simulink model "wave_4"  (Simulink 7.4)
settings: Solver=ode23tb  StartTime=0.0  StopTime=.5  RelTol=1e-3
PreLoadFcn:
  | load gauss_fir;  % pulse shaping coefficients
InitFcn:
  | Ts=1e-4;    % set this to control simulation speed, mainly for wave visualization
  | Line_Length=0.05; % meters
libraries: powerlib x208, simulink x2, dspsrcs4 x1
(part 2 of 2)

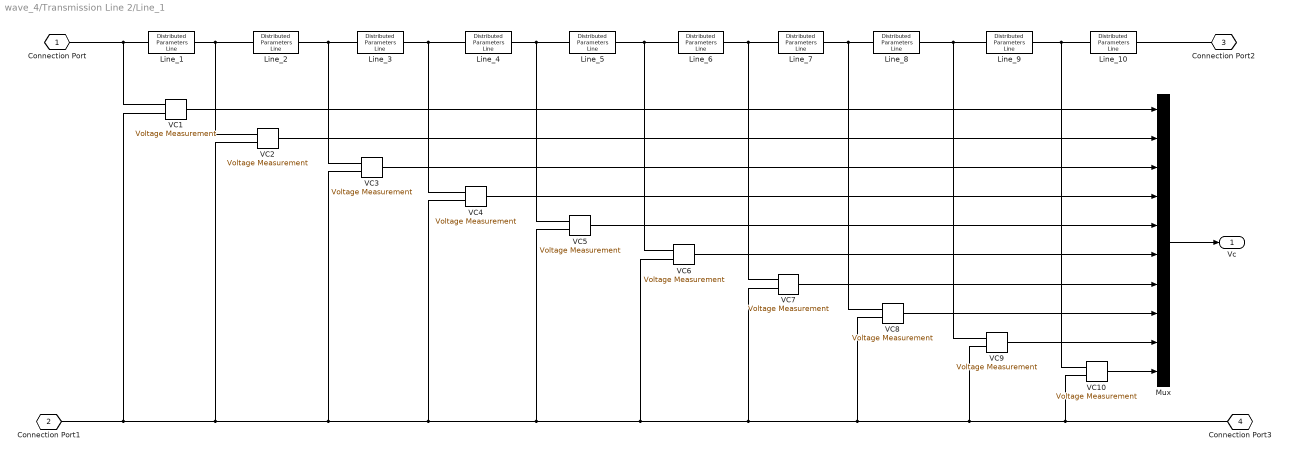
== system wave_4/Transmission Line 2/Line_1 ==
  Line_1 : powerlib/Elements/Distributed Parameters Line  DialogController=POWERSYS.PowerSysDialog  SystemSampleTime=-1  Phases=1  Frequency=60  Resistance=R(1)*1000  Inductance=L(1)*1000  Capacitance=C(1)*1000  Length=Len/(10*1000); % 10 sections in this subsystem  x1=[0 0;0.0002 0;0.0004 0;0.0006 0;0.0008 0;0.001 0]  x2=[0 0;0.0002 0;0.0004 0;0.0006 0;0.0008 0;0.001 0]  x3=[0 0;0.0002 0;0.0004 0;0.0006 0;0.0008 0;0.001 0]  x4=[0 0;0.0002 0;0.0004 0;0.0006 0;0.0008 0;0.001 0]  x5=0.001  Measurements=None
  Line_10 : powerlib/Elements/Distributed Parameters Line  DialogController=POWERSYS.PowerSysDialog  SystemSampleTime=-1  Phases=1  Frequency=60  Resistance=R(10)*1000  Inductance=L(10)*1000  Capacitance=C(10)*1000  Length=Len/(10*1000); % 10 sections in this subsystem  x1=[0 0;0.0002 0;0.0004 0;0.0006 0;0.0008 0;0.001 0]  x2=[0 0;0.0002 0;0.0004 0;0.0006 0;0.0008 0;0.001 0]  x3=[0 0;0.0002 0;0.0004 0;0.0006 0;0.0008 0;0.001 0]  x4=[0 0;0.0002 0;0.0004 0;0.0006 0;0.0008 0;0.001 0]  x5=0.001  Measurements=None
  Line_2 : powerlib/Elements/Distributed Parameters Line  DialogController=POWERSYS.PowerSysDialog  SystemSampleTime=-1  Phases=1  Frequency=60  Resistance=R(2)*1000  Inductance=L(2)*1000  Capacitance=C(2)*1000  Length=Len/(10*1000); % 10 sections in this subsystem  x1=[0 0;0.0002 0;0.0004 0;0.0006 0;0.0008 0;0.001 0]  x2=[0 0;0.0002 0;0.0004 0;0.0006 0;0.0008 0;0.001 0]  x3=[0 0;0.0002 0;0.0004 0;0.0006 0;0.0008 0;0.001 0]  x4=[0 0;0.0002 0;0.0004 0;0.0006 0;0.0008 0;0.001 0]  x5=0.001  Measurements=None
  Line_3 : powerlib/Elements/Distributed Parameters Line  DialogController=POWERSYS.PowerSysDialog  SystemSampleTime=-1  Phases=1  Frequency=60  Resistance=R(3)*1000  Inductance=L(3)*1000  Capacitance=C(3)*1000  Length=Len/(10*1000); % 10 sections in this subsystem  x1=[0 0;0.0002 0;0.0004 0;0.0006 0;0.0008 0;0.001 0]  x2=[0 0;0.0002 0;0.0004 0;0.0006 0;0.0008 0;0.001 0]  x3=[0 0;0.0002 0;0.0004 0;0.0006 0;0.0008 0;0.001 0]  x4=[0 0;0.0002 0;0.0004 0;0.0006 0;0.0008 0;0.001 0]  x5=0.001  Measurements=None
  Line_4 : powerlib/Elements/Distributed Parameters Line  DialogController=POWERSYS.PowerSysDialog  SystemSampleTime=-1  Phases=1  Frequency=60  Resistance=R(4)*1000  Inductance=L(4)*1000  Capacitance=C(4)*1000  Length=Len/(10*1000); % 10 sections in this subsystem  x1=[0 0;0.0002 0;0.0004 0;0.0006 0;0.0008 0;0.001 0]  x2=[0 0;0.0002 0;0.0004 0;0.0006 0;0.0008 0;0.001 0]  x3=[0 0;0.0002 0;0.0004 0;0.0006 0;0.0008 0;0.001 0]  x4=[0 0;0.0002 0;0.0004 0;0.0006 0;0.0008 0;0.001 0]  x5=0.001  Measurements=None
  Line_5 : powerlib/Elements/Distributed Parameters Line  DialogController=POWERSYS.PowerSysDialog  SystemSampleTime=-1  Phases=1  Frequency=60  Resistance=R(5)*1000  Inductance=L(5)*1000  Capacitance=C(5)*1000  Length=Len/(10*1000); % 10 sections in this subsystem  x1=[0 0;0.0002 0;0.0004 0;0.0006 0;0.0008 0;0.001 0]  x2=[0 0;0.0002 0;0.0004 0;0.0006 0;0.0008 0;0.001 0]  x3=[0 0;0.0002 0;0.0004 0;0.0006 0;0.0008 0;0.001 0]  x4=[0 0;0.0002 0;0.0004 0;0.0006 0;0.0008 0;0.001 0]  x5=0.001  Measurements=None
  Line_6 : powerlib/Elements/Distributed Parameters Line  DialogController=POWERSYS.PowerSysDialog  SystemSampleTime=-1  Phases=1  Frequency=60  Resistance=R(6)*1000  Inductance=L(6)*1000  Capacitance=C(6)*1000  Length=Len/(10*1000); % 10 sections in this subsystem  x1=[0 0;0.0002 0;0.0004 0;0.0006 0;0.0008 0;0.001 0]  x2=[0 0;0.0002 0;0.0004 0;0.0006 0;0.0008 0;0.001 0]  x3=[0 0;0.0002 0;0.0004 0;0.0006 0;0.0008 0;0.001 0]  x4=[0 0;0.0002 0;0.0004 0;0.0006 0;0.0008 0;0.001 0]  x5=0.001  Measurements=None
  Line_7 : powerlib/Elements/Distributed Parameters Line  DialogController=POWERSYS.PowerSysDialog  SystemSampleTime=-1  Phases=1  Frequency=60  Resistance=R(7)*1000  Inductance=L(7)*1000  Capacitance=C(7)*1000  Length=Len/(10*1000); % 10 sections in this subsystem  x1=[0 0;0.0002 0;0.0004 0;0.0006 0;0.0008 0;0.001 0]  x2=[0 0;0.0002 0;0.0004 0;0.0006 0;0.0008 0;0.001 0]  x3=[0 0;0.0002 0;0.0004 0;0.0006 0;0.0008 0;0.001 0]  x4=[0 0;0.0002 0;0.0004 0;0.0006 0;0.0008 0;0.001 0]  x5=0.001  Measurements=None
  Line_8 : powerlib/Elements/Distributed Parameters Line  DialogController=POWERSYS.PowerSysDialog  SystemSampleTime=-1  Phases=1  Frequency=60  Resistance=R(8)*1000  Inductance=L(8)*1000  Capacitance=C(8)*1000  Length=Len/(10*1000); % 10 sections in this subsystem  x1=[0 0;0.0002 0;0.0004 0;0.0006 0;0.0008 0;0.001 0]  x2=[0 0;0.0002 0;0.0004 0;0.0006 0;0.0008 0;0.001 0]  x3=[0 0;0.0002 0;0.0004 0;0.0006 0;0.0008 0;0.001 0]  x4=[0 0;0.0002 0;0.0004 0;0.0006 0;0.0008 0;0.001 0]  x5=0.001  Measurements=None
  Line_9 : powerlib/Elements/Distributed Parameters Line  DialogController=POWERSYS.PowerSysDialog  SystemSampleTime=-1  Phases=1  Frequency=60  Resistance=R(9)*1000  Inductance=L(9)*1000  Capacitance=C(9)*1000  Length=Len/(10*1000); % 10 sections in this subsystem  x1=[0 0;0.0002 0;0.0004 0;0.0006 0;0.0008 0;0.001 0]  x2=[0 0;0.0002 0;0.0004 0;0.0006 0;0.0008 0;0.001 0]  x3=[0 0;0.0002 0;0.0004 0;0.0006 0;0.0008 0;0.001 0]  x4=[0 0;0.0002 0;0.0004 0;0.0006 0;0.0008 0;0.001 0]  x5=0.001  Measurements=None
  Mux : Mux  Inputs=10
  VC{1..10} (10 alike) : powerlib/Measurements/Voltage Measurement  DialogController=POWERSYS.PowerSysDialog  SystemSampleTime=-1  PhasorSimulation=off  OutputType=Complex  PSBequivalent=0
  Connection Port : PMIOPort  Tag=PMCPort  Port=1  Side=Left
  Connection Port1 : PMIOPort  Tag=PMCPort  Port=2  Side=Left
  Connection Port2 : PMIOPort  Tag=PMCPort  Port=3  Side=Right
  Connection Port3 : PMIOPort  Tag=PMCPort  Port=4  Side=Right
  Vc : Outport  OutDataType=fixdt(1, 16)  OutScaling=2^0
  wires:
  Mux/1 -> Vc/1
  VC2/1 -> Mux/2
  VC3/1 -> Mux/3
  VC4/1 -> Mux/4
  VC5/1 -> Mux/5
  VC6/1 -> Mux/6
  VC7/1 -> Mux/7
  VC8/1 -> Mux/8
  VC9/1 -> Mux/9
  VC10/1 -> Mux/10
  VC1/1 -> Mux/1
  connections:
  VC10/LConn1 -- Line_10/LConn1 -- Line_9/RConn1
  VC9/LConn1 -- Line_9/LConn1 -- Line_8/RConn1
  VC8/LConn1 -- Line_8/LConn1 -- Line_7/RConn1
  VC7/LConn1 -- Line_7/LConn1 -- Line_6/RConn1
  VC6/LConn1 -- Line_6/LConn1 -- Line_5/RConn1
  VC5/LConn1 -- Line_5/LConn1 -- Line_4/RConn1
  VC4/LConn1 -- Line_4/LConn1 -- Line_3/RConn1
  VC3/LConn1 -- Line_3/LConn1 -- Line_2/RConn1
  VC2/LConn1 -- Line_2/LConn1 -- Line_1/RConn1
  VC1/LConn1 -- Line_1/LConn1 -- Connection Port/RConn1
  Line_10/RConn1 -- Connection Port2/RConn1
  VC1/LConn2 -- VC2/LConn2 -- VC3/LConn2 -- VC4/LConn2 -- VC5/LConn2 -- VC6/LConn2 -- VC7/LConn2 -- VC8/LConn2 -- VC9/LConn2 -- VC10/LConn2 -- Connection Port3/RConn1 -- Connection Port1/RConn1

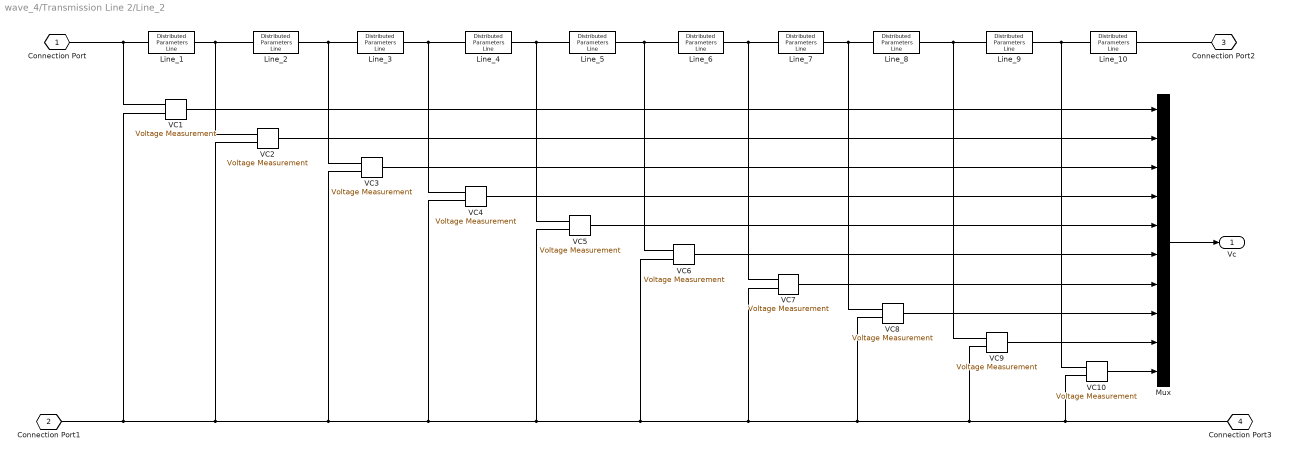
== system wave_4/Transmission Line 2/Line_2 ==
  Line_1 : powerlib/Elements/Distributed Parameters Line  DialogController=POWERSYS.PowerSysDialog  SystemSampleTime=-1  Phases=1  Frequency=60  Resistance=R(1)*1000  Inductance=L(1)*1000  Capacitance=C(1)*1000  Length=Len/(10*1000); % 10 sections in this subsystem  x1=[0 0;0.0002 0;0.0004 0;0.0006 0;0.0008 0;0.001 0]  x2=[0 0;0.0002 0;0.0004 0;0.0006 0;0.0008 0;0.001 0]  x3=[0 0;0.0002 0;0.0004 0;0.0006 0;0.0008 0;0.001 0]  x4=[0 0;0.0002 0;0.0004 0;0.0006 0;0.0008 0;0.001 0]  x5=0.001  Measurements=None
  Line_10 : powerlib/Elements/Distributed Parameters Line  DialogController=POWERSYS.PowerSysDialog  SystemSampleTime=-1  Phases=1  Frequency=60  Resistance=R(10)*1000  Inductance=L(10)*1000  Capacitance=C(10)*1000  Length=Len/(10*1000); % 10 sections in this subsystem  x1=[0 0;0.0002 0;0.0004 0;0.0006 0;0.0008 0;0.001 0]  x2=[0 0;0.0002 0;0.0004 0;0.0006 0;0.0008 0;0.001 0]  x3=[0 0;0.0002 0;0.0004 0;0.0006 0;0.0008 0;0.001 0]  x4=[0 0;0.0002 0;0.0004 0;0.0006 0;0.0008 0;0.001 0]  x5=0.001  Measurements=None
  Line_2 : powerlib/Elements/Distributed Parameters Line  DialogController=POWERSYS.PowerSysDialog  SystemSampleTime=-1  Phases=1  Frequency=60  Resistance=R(2)*1000  Inductance=L(2)*1000  Capacitance=C(2)*1000  Length=Len/(10*1000); % 10 sections in this subsystem  x1=[0 0;0.0002 0;0.0004 0;0.0006 0;0.0008 0;0.001 0]  x2=[0 0;0.0002 0;0.0004 0;0.0006 0;0.0008 0;0.001 0]  x3=[0 0;0.0002 0;0.0004 0;0.0006 0;0.0008 0;0.001 0]  x4=[0 0;0.0002 0;0.0004 0;0.0006 0;0.0008 0;0.001 0]  x5=0.001  Measurements=None
  Line_3 : powerlib/Elements/Distributed Parameters Line  DialogController=POWERSYS.PowerSysDialog  SystemSampleTime=-1  Phases=1  Frequency=60  Resistance=R(3)*1000  Inductance=L(3)*1000  Capacitance=C(3)*1000  Length=Len/(10*1000); % 10 sections in this subsystem  x1=[0 0;0.0002 0;0.0004 0;0.0006 0;0.0008 0;0.001 0]  x2=[0 0;0.0002 0;0.0004 0;0.0006 0;0.0008 0;0.001 0]  x3=[0 0;0.0002 0;0.0004 0;0.0006 0;0.0008 0;0.001 0]  x4=[0 0;0.0002 0;0.0004 0;0.0006 0;0.0008 0;0.001 0]  x5=0.001  Measurements=None
  Line_4 : powerlib/Elements/Distributed Parameters Line  DialogController=POWERSYS.PowerSysDialog  SystemSampleTime=-1  Phases=1  Frequency=60  Resistance=R(4)*1000  Inductance=L(4)*1000  Capacitance=C(4)*1000  Length=Len/(10*1000); % 10 sections in this subsystem  x1=[0 0;0.0002 0;0.0004 0;0.0006 0;0.0008 0;0.001 0]  x2=[0 0;0.0002 0;0.0004 0;0.0006 0;0.0008 0;0.001 0]  x3=[0 0;0.0002 0;0.0004 0;0.0006 0;0.0008 0;0.001 0]  x4=[0 0;0.0002 0;0.0004 0;0.0006 0;0.0008 0;0.001 0]  x5=0.001  Measurements=None
  Line_5 : powerlib/Elements/Distributed Parameters Line  DialogController=POWERSYS.PowerSysDialog  SystemSampleTime=-1  Phases=1  Frequency=60  Resistance=R(5)*1000  Inductance=L(5)*1000  Capacitance=C(5)*1000  Length=Len/(10*1000); % 10 sections in this subsystem  x1=[0 0;0.0002 0;0.0004 0;0.0006 0;0.0008 0;0.001 0]  x2=[0 0;0.0002 0;0.0004 0;0.0006 0;0.0008 0;0.001 0]  x3=[0 0;0.0002 0;0.0004 0;0.0006 0;0.0008 0;0.001 0]  x4=[0 0;0.0002 0;0.0004 0;0.0006 0;0.0008 0;0.001 0]  x5=0.001  Measurements=None
  Line_6 : powerlib/Elements/Distributed Parameters Line  DialogController=POWERSYS.PowerSysDialog  SystemSampleTime=-1  Phases=1  Frequency=60  Resistance=R(6)*1000  Inductance=L(6)*1000  Capacitance=C(6)*1000  Length=Len/(10*1000); % 10 sections in this subsystem  x1=[0 0;0.0002 0;0.0004 0;0.0006 0;0.0008 0;0.001 0]  x2=[0 0;0.0002 0;0.0004 0;0.0006 0;0.0008 0;0.001 0]  x3=[0 0;0.0002 0;0.0004 0;0.0006 0;0.0008 0;0.001 0]  x4=[0 0;0.0002 0;0.0004 0;0.0006 0;0.0008 0;0.001 0]  x5=0.001  Measurements=None
  Line_7 : powerlib/Elements/Distributed Parameters Line  DialogController=POWERSYS.PowerSysDialog  SystemSampleTime=-1  Phases=1  Frequency=60  Resistance=R(7)*1000  Inductance=L(7)*1000  Capacitance=C(7)*1000  Length=Len/(10*1000); % 10 sections in this subsystem  x1=[0 0;0.0002 0;0.0004 0;0.0006 0;0.0008 0;0.001 0]  x2=[0 0;0.0002 0;0.0004 0;0.0006 0;0.0008 0;0.001 0]  x3=[0 0;0.0002 0;0.0004 0;0.0006 0;0.0008 0;0.001 0]  x4=[0 0;0.0002 0;0.0004 0;0.0006 0;0.0008 0;0.001 0]  x5=0.001  Measurements=None
  Line_8 : powerlib/Elements/Distributed Parameters Line  DialogController=POWERSYS.PowerSysDialog  SystemSampleTime=-1  Phases=1  Frequency=60  Resistance=R(8)*1000  Inductance=L(8)*1000  Capacitance=C(8)*1000  Length=Len/(10*1000); % 10 sections in this subsystem  x1=[0 0;0.0002 0;0.0004 0;0.0006 0;0.0008 0;0.001 0]  x2=[0 0;0.0002 0;0.0004 0;0.0006 0;0.0008 0;0.001 0]  x3=[0 0;0.0002 0;0.0004 0;0.0006 0;0.0008 0;0.001 0]  x4=[0 0;0.0002 0;0.0004 0;0.0006 0;0.0008 0;0.001 0]  x5=0.001  Measurements=None
  Line_9 : powerlib/Elements/Distributed Parameters Line  DialogController=POWERSYS.PowerSysDialog  SystemSampleTime=-1  Phases=1  Frequency=60  Resistance=R(9)*1000  Inductance=L(9)*1000  Capacitance=C(9)*1000  Length=Len/(10*1000); % 10 sections in this subsystem  x1=[0 0;0.0002 0;0.0004 0;0.0006 0;0.0008 0;0.001 0]  x2=[0 0;0.0002 0;0.0004 0;0.0006 0;0.0008 0;0.001 0]  x3=[0 0;0.0002 0;0.0004 0;0.0006 0;0.0008 0;0.001 0]  x4=[0 0;0.0002 0;0.0004 0;0.0006 0;0.0008 0;0.001 0]  x5=0.001  Measurements=None
  Mux : Mux  Inputs=10
  VC{1..10} (10 alike) : powerlib/Measurements/Voltage Measurement  DialogController=POWERSYS.PowerSysDialog  SystemSampleTime=-1  PhasorSimulation=off  OutputType=Complex  PSBequivalent=0
  Connection Port : PMIOPort  Tag=PMCPort  Port=1  Side=Left
  Connection Port1 : PMIOPort  Tag=PMCPort  Port=2  Side=Left
  Connection Port2 : PMIOPort  Tag=PMCPort  Port=3  Side=Right
  Connection Port3 : PMIOPort  Tag=PMCPort  Port=4  Side=Right
  Vc : Outport  OutDataType=fixdt(1, 16)  OutScaling=2^0
  wires:
  VC1/1 -> Mux/1
  VC10/1 -> Mux/10
  VC9/1 -> Mux/9
  VC8/1 -> Mux/8
  VC7/1 -> Mux/7
  VC6/1 -> Mux/6
  VC5/1 -> Mux/5
  VC4/1 -> Mux/4
  VC3/1 -> Mux/3
  VC2/1 -> Mux/2
  Mux/1 -> Vc/1
  connections:
  Connection Port1/RConn1 -- Connection Port3/RConn1 -- VC10/LConn2 -- VC9/LConn2 -- VC8/LConn2 -- VC7/LConn2 -- VC6/LConn2 -- VC5/LConn2 -- VC4/LConn2 -- VC3/LConn2 -- VC2/LConn2 -- VC1/LConn2
  Line_10/RConn1 -- Connection Port2/RConn1
  Connection Port/RConn1 -- Line_1/LConn1 -- VC1/LConn1
  Line_1/RConn1 -- Line_2/LConn1 -- VC2/LConn1
  Line_2/RConn1 -- Line_3/LConn1 -- VC3/LConn1
  Line_3/RConn1 -- Line_4/LConn1 -- VC4/LConn1
  Line_4/RConn1 -- Line_5/LConn1 -- VC5/LConn1
  Line_5/RConn1 -- Line_6/LConn1 -- VC6/LConn1
  Line_6/RConn1 -- Line_7/LConn1 -- VC7/LConn1
  Line_7/RConn1 -- Line_8/LConn1 -- VC8/LConn1
  Line_8/RConn1 -- Line_9/LConn1 -- VC9/LConn1
  Line_9/RConn1 -- Line_10/LConn1 -- VC10/LConn1

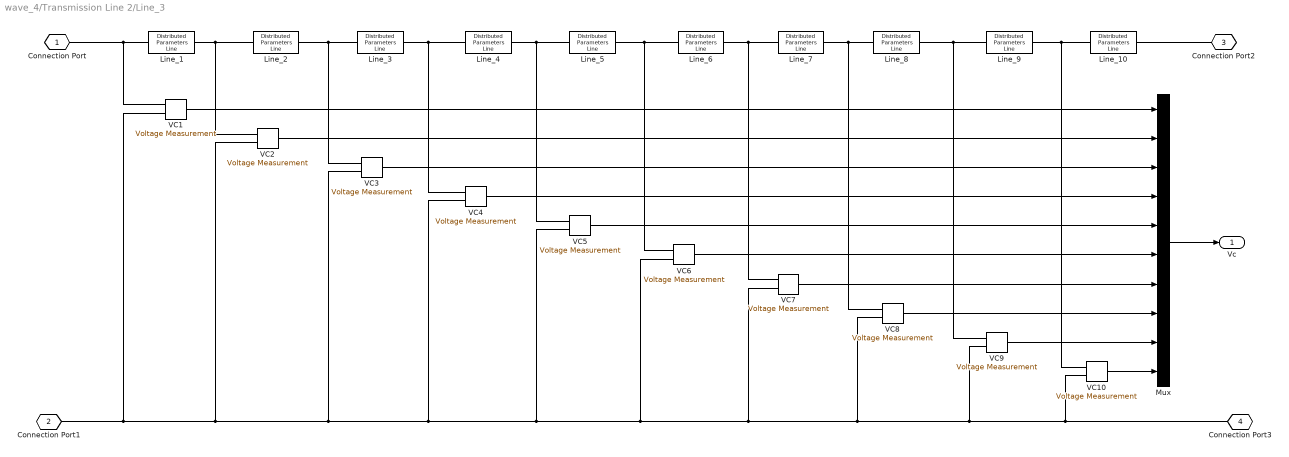
== system wave_4/Transmission Line 2/Line_3 ==
  Line_1 : powerlib/Elements/Distributed Parameters Line  DialogController=POWERSYS.PowerSysDialog  SystemSampleTime=-1  Phases=1  Frequency=60  Resistance=R(1)*1000  Inductance=L(1)*1000  Capacitance=C(1)*1000  Length=Len/(10*1000); % 10 sections in this subsystem  x1=[0 0;0.0002 0;0.0004 0;0.0006 0;0.0008 0;0.001 0]  x2=[0 0;0.0002 0;0.0004 0;0.0006 0;0.0008 0;0.001 0]  x3=[0 0;0.0002 0;0.0004 0;0.0006 0;0.0008 0;0.001 0]  x4=[0 0;0.0002 0;0.0004 0;0.0006 0;0.0008 0;0.001 0]  x5=0.001  Measurements=None
  Line_10 : powerlib/Elements/Distributed Parameters Line  DialogController=POWERSYS.PowerSysDialog  SystemSampleTime=-1  Phases=1  Frequency=60  Resistance=R(10)*1000  Inductance=L(10)*1000  Capacitance=C(10)*1000  Length=Len/(10*1000); % 10 sections in this subsystem  x1=[0 0;0.0002 0;0.0004 0;0.0006 0;0.0008 0;0.001 0]  x2=[0 0;0.0002 0;0.0004 0;0.0006 0;0.0008 0;0.001 0]  x3=[0 0;0.0002 0;0.0004 0;0.0006 0;0.0008 0;0.001 0]  x4=[0 0;0.0002 0;0.0004 0;0.0006 0;0.0008 0;0.001 0]  x5=0.001  Measurements=None
  Line_2 : powerlib/Elements/Distributed Parameters Line  DialogController=POWERSYS.PowerSysDialog  SystemSampleTime=-1  Phases=1  Frequency=60  Resistance=R(2)*1000  Inductance=L(2)*1000  Capacitance=C(2)*1000  Length=Len/(10*1000); % 10 sections in this subsystem  x1=[0 0;0.0002 0;0.0004 0;0.0006 0;0.0008 0;0.001 0]  x2=[0 0;0.0002 0;0.0004 0;0.0006 0;0.0008 0;0.001 0]  x3=[0 0;0.0002 0;0.0004 0;0.0006 0;0.0008 0;0.001 0]  x4=[0 0;0.0002 0;0.0004 0;0.0006 0;0.0008 0;0.001 0]  x5=0.001  Measurements=None
  Line_3 : powerlib/Elements/Distributed Parameters Line  DialogController=POWERSYS.PowerSysDialog  SystemSampleTime=-1  Phases=1  Frequency=60  Resistance=R(3)*1000  Inductance=L(3)*1000  Capacitance=C(3)*1000  Length=Len/(10*1000); % 10 sections in this subsystem  x1=[0 0;0.0002 0;0.0004 0;0.0006 0;0.0008 0;0.001 0]  x2=[0 0;0.0002 0;0.0004 0;0.0006 0;0.0008 0;0.001 0]  x3=[0 0;0.0002 0;0.0004 0;0.0006 0;0.0008 0;0.001 0]  x4=[0 0;0.0002 0;0.0004 0;0.0006 0;0.0008 0;0.001 0]  x5=0.001  Measurements=None
  Line_4 : powerlib/Elements/Distributed Parameters Line  DialogController=POWERSYS.PowerSysDialog  SystemSampleTime=-1  Phases=1  Frequency=60  Resistance=R(4)*1000  Inductance=L(4)*1000  Capacitance=C(4)*1000  Length=Len/(10*1000); % 10 sections in this subsystem  x1=[0 0;0.0002 0;0.0004 0;0.0006 0;0.0008 0;0.001 0]  x2=[0 0;0.0002 0;0.0004 0;0.0006 0;0.0008 0;0.001 0]  x3=[0 0;0.0002 0;0.0004 0;0.0006 0;0.0008 0;0.001 0]  x4=[0 0;0.0002 0;0.0004 0;0.0006 0;0.0008 0;0.001 0]  x5=0.001  Measurements=None
  Line_5 : powerlib/Elements/Distributed Parameters Line  DialogController=POWERSYS.PowerSysDialog  SystemSampleTime=-1  Phases=1  Frequency=60  Resistance=R(5)*1000  Inductance=L(5)*1000  Capacitance=C(5)*1000  Length=Len/(10*1000); % 10 sections in this subsystem  x1=[0 0;0.0002 0;0.0004 0;0.0006 0;0.0008 0;0.001 0]  x2=[0 0;0.0002 0;0.0004 0;0.0006 0;0.0008 0;0.001 0]  x3=[0 0;0.0002 0;0.0004 0;0.0006 0;0.0008 0;0.001 0]  x4=[0 0;0.0002 0;0.0004 0;0.0006 0;0.0008 0;0.001 0]  x5=0.001  Measurements=None
  Line_6 : powerlib/Elements/Distributed Parameters Line  DialogController=POWERSYS.PowerSysDialog  SystemSampleTime=-1  Phases=1  Frequency=60  Resistance=R(6)*1000  Inductance=L(6)*1000  Capacitance=C(6)*1000  Length=Len/(10*1000); % 10 sections in this subsystem  x1=[0 0;0.0002 0;0.0004 0;0.0006 0;0.0008 0;0.001 0]  x2=[0 0;0.0002 0;0.0004 0;0.0006 0;0.0008 0;0.001 0]  x3=[0 0;0.0002 0;0.0004 0;0.0006 0;0.0008 0;0.001 0]  x4=[0 0;0.0002 0;0.0004 0;0.0006 0;0.0008 0;0.001 0]  x5=0.001  Measurements=None
  Line_7 : powerlib/Elements/Distributed Parameters Line  DialogController=POWERSYS.PowerSysDialog  SystemSampleTime=-1  Phases=1  Frequency=60  Resistance=R(7)*1000  Inductance=L(7)*1000  Capacitance=C(7)*1000  Length=Len/(10*1000); % 10 sections in this subsystem  x1=[0 0;0.0002 0;0.0004 0;0.0006 0;0.0008 0;0.001 0]  x2=[0 0;0.0002 0;0.0004 0;0.0006 0;0.0008 0;0.001 0]  x3=[0 0;0.0002 0;0.0004 0;0.0006 0;0.0008 0;0.001 0]  x4=[0 0;0.0002 0;0.0004 0;0.0006 0;0.0008 0;0.001 0]  x5=0.001  Measurements=None
  Line_8 : powerlib/Elements/Distributed Parameters Line  DialogController=POWERSYS.PowerSysDialog  SystemSampleTime=-1  Phases=1  Frequency=60  Resistance=R(8)*1000  Inductance=L(8)*1000  Capacitance=C(8)*1000  Length=Len/(10*1000); % 10 sections in this subsystem  x1=[0 0;0.0002 0;0.0004 0;0.0006 0;0.0008 0;0.001 0]  x2=[0 0;0.0002 0;0.0004 0;0.0006 0;0.0008 0;0.001 0]  x3=[0 0;0.0002 0;0.0004 0;0.0006 0;0.0008 0;0.001 0]  x4=[0 0;0.0002 0;0.0004 0;0.0006 0;0.0008 0;0.001 0]  x5=0.001  Measurements=None
  Line_9 : powerlib/Elements/Distributed Parameters Line  DialogController=POWERSYS.PowerSysDialog  SystemSampleTime=-1  Phases=1  Frequency=60  Resistance=R(9)*1000  Inductance=L(9)*1000  Capacitance=C(9)*1000  Length=Len/(10*1000); % 10 sections in this subsystem  x1=[0 0;0.0002 0;0.0004 0;0.0006 0;0.0008 0;0.001 0]  x2=[0 0;0.0002 0;0.0004 0;0.0006 0;0.0008 0;0.001 0]  x3=[0 0;0.0002 0;0.0004 0;0.0006 0;0.0008 0;0.001 0]  x4=[0 0;0.0002 0;0.0004 0;0.0006 0;0.0008 0;0.001 0]  x5=0.001  Measurements=None
  Mux : Mux  Inputs=10
  VC{1..10} (10 alike) : powerlib/Measurements/Voltage Measurement  DialogController=POWERSYS.PowerSysDialog  SystemSampleTime=-1  PhasorSimulation=off  OutputType=Complex  PSBequivalent=0
  Connection Port : PMIOPort  Tag=PMCPort  Port=1  Side=Left
  Connection Port1 : PMIOPort  Tag=PMCPort  Port=2  Side=Left
  Connection Port2 : PMIOPort  Tag=PMCPort  Port=3  Side=Right
  Connection Port3 : PMIOPort  Tag=PMCPort  Port=4  Side=Right
  Vc : Outport  OutDataType=fixdt(1, 16)  OutScaling=2^0
  wires:
  Mux/1 -> Vc/1
  VC2/1 -> Mux/2
  VC3/1 -> Mux/3
  VC4/1 -> Mux/4
  VC5/1 -> Mux/5
  VC6/1 -> Mux/6
  VC7/1 -> Mux/7
  VC8/1 -> Mux/8
  VC9/1 -> Mux/9
  VC10/1 -> Mux/10
  VC1/1 -> Mux/1
  connections:
  VC10/LConn1 -- Line_10/LConn1 -- Line_9/RConn1
  VC9/LConn1 -- Line_9/LConn1 -- Line_8/RConn1
  VC8/LConn1 -- Line_8/LConn1 -- Line_7/RConn1
  VC7/LConn1 -- Line_7/LConn1 -- Line_6/RConn1
  VC6/LConn1 -- Line_6/LConn1 -- Line_5/RConn1
  VC5/LConn1 -- Line_5/LConn1 -- Line_4/RConn1
  VC4/LConn1 -- Line_4/LConn1 -- Line_3/RConn1
  VC3/LConn1 -- Line_3/LConn1 -- Line_2/RConn1
  VC2/LConn1 -- Line_2/LConn1 -- Line_1/RConn1
  VC1/LConn1 -- Line_1/LConn1 -- Connection Port/RConn1
  Line_10/RConn1 -- Connection Port2/RConn1
  VC1/LConn2 -- VC2/LConn2 -- VC3/LConn2 -- VC4/LConn2 -- VC5/LConn2 -- VC6/LConn2 -- VC7/LConn2 -- VC8/LConn2 -- VC9/LConn2 -- VC10/LConn2 -- Connection Port3/RConn1 -- Connection Port1/RConn1

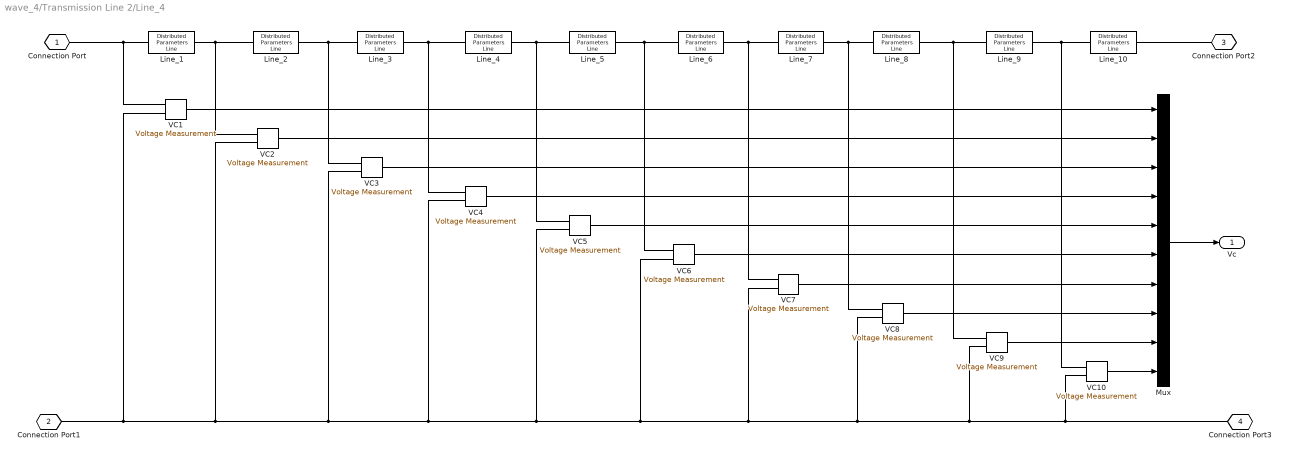
== system wave_4/Transmission Line 2/Line_4 ==
  Line_1 : powerlib/Elements/Distributed Parameters Line  DialogController=POWERSYS.PowerSysDialog  SystemSampleTime=-1  Phases=1  Frequency=60  Resistance=R(1)*1000  Inductance=L(1)*1000  Capacitance=C(1)*1000  Length=Len/(10*1000); % 10 sections in this subsystem  x1=[0 0;0.0002 0;0.0004 0;0.0006 0;0.0008 0;0.001 0]  x2=[0 0;0.0002 0;0.0004 0;0.0006 0;0.0008 0;0.001 0]  x3=[0 0;0.0002 0;0.0004 0;0.0006 0;0.0008 0;0.001 0]  x4=[0 0;0.0002 0;0.0004 0;0.0006 0;0.0008 0;0.001 0]  x5=0.001  Measurements=None
  Line_10 : powerlib/Elements/Distributed Parameters Line  DialogController=POWERSYS.PowerSysDialog  SystemSampleTime=-1  Phases=1  Frequency=60  Resistance=R(10)*1000  Inductance=L(10)*1000  Capacitance=C(10)*1000  Length=Len/(10*1000); % 10 sections in this subsystem  x1=[0 0;0.0002 0;0.0004 0;0.0006 0;0.0008 0;0.001 0]  x2=[0 0;0.0002 0;0.0004 0;0.0006 0;0.0008 0;0.001 0]  x3=[0 0;0.0002 0;0.0004 0;0.0006 0;0.0008 0;0.001 0]  x4=[0 0;0.0002 0;0.0004 0;0.0006 0;0.0008 0;0.001 0]  x5=0.001  Measurements=None
  Line_2 : powerlib/Elements/Distributed Parameters Line  DialogController=POWERSYS.PowerSysDialog  SystemSampleTime=-1  Phases=1  Frequency=60  Resistance=R(2)*1000  Inductance=L(2)*1000  Capacitance=C(2)*1000  Length=Len/(10*1000); % 10 sections in this subsystem  x1=[0 0;0.0002 0;0.0004 0;0.0006 0;0.0008 0;0.001 0]  x2=[0 0;0.0002 0;0.0004 0;0.0006 0;0.0008 0;0.001 0]  x3=[0 0;0.0002 0;0.0004 0;0.0006 0;0.0008 0;0.001 0]  x4=[0 0;0.0002 0;0.0004 0;0.0006 0;0.0008 0;0.001 0]  x5=0.001  Measurements=None
  Line_3 : powerlib/Elements/Distributed Parameters Line  DialogController=POWERSYS.PowerSysDialog  SystemSampleTime=-1  Phases=1  Frequency=60  Resistance=R(3)*1000  Inductance=L(3)*1000  Capacitance=C(3)*1000  Length=Len/(10*1000); % 10 sections in this subsystem  x1=[0 0;0.0002 0;0.0004 0;0.0006 0;0.0008 0;0.001 0]  x2=[0 0;0.0002 0;0.0004 0;0.0006 0;0.0008 0;0.001 0]  x3=[0 0;0.0002 0;0.0004 0;0.0006 0;0.0008 0;0.001 0]  x4=[0 0;0.0002 0;0.0004 0;0.0006 0;0.0008 0;0.001 0]  x5=0.001  Measurements=None
  Line_4 : powerlib/Elements/Distributed Parameters Line  DialogController=POWERSYS.PowerSysDialog  SystemSampleTime=-1  Phases=1  Frequency=60  Resistance=R(4)*1000  Inductance=L(4)*1000  Capacitance=C(4)*1000  Length=Len/(10*1000); % 10 sections in this subsystem  x1=[0 0;0.0002 0;0.0004 0;0.0006 0;0.0008 0;0.001 0]  x2=[0 0;0.0002 0;0.0004 0;0.0006 0;0.0008 0;0.001 0]  x3=[0 0;0.0002 0;0.0004 0;0.0006 0;0.0008 0;0.001 0]  x4=[0 0;0.0002 0;0.0004 0;0.0006 0;0.0008 0;0.001 0]  x5=0.001  Measurements=None
  Line_5 : powerlib/Elements/Distributed Parameters Line  DialogController=POWERSYS.PowerSysDialog  SystemSampleTime=-1  Phases=1  Frequency=60  Resistance=R(5)*1000  Inductance=L(5)*1000  Capacitance=C(5)*1000  Length=Len/(10*1000); % 10 sections in this subsystem  x1=[0 0;0.0002 0;0.0004 0;0.0006 0;0.0008 0;0.001 0]  x2=[0 0;0.0002 0;0.0004 0;0.0006 0;0.0008 0;0.001 0]  x3=[0 0;0.0002 0;0.0004 0;0.0006 0;0.0008 0;0.001 0]  x4=[0 0;0.0002 0;0.0004 0;0.0006 0;0.0008 0;0.001 0]  x5=0.001  Measurements=None
  Line_6 : powerlib/Elements/Distributed Parameters Line  DialogController=POWERSYS.PowerSysDialog  SystemSampleTime=-1  Phases=1  Frequency=60  Resistance=R(6)*1000  Inductance=L(6)*1000  Capacitance=C(6)*1000  Length=Len/(10*1000); % 10 sections in this subsystem  x1=[0 0;0.0002 0;0.0004 0;0.0006 0;0.0008 0;0.001 0]  x2=[0 0;0.0002 0;0.0004 0;0.0006 0;0.0008 0;0.001 0]  x3=[0 0;0.0002 0;0.0004 0;0.0006 0;0.0008 0;0.001 0]  x4=[0 0;0.0002 0;0.0004 0;0.0006 0;0.0008 0;0.001 0]  x5=0.001  Measurements=None
  Line_7 : powerlib/Elements/Distributed Parameters Line  DialogController=POWERSYS.PowerSysDialog  SystemSampleTime=-1  Phases=1  Frequency=60  Resistance=R(7)*1000  Inductance=L(7)*1000  Capacitance=C(7)*1000  Length=Len/(10*1000); % 10 sections in this subsystem  x1=[0 0;0.0002 0;0.0004 0;0.0006 0;0.0008 0;0.001 0]  x2=[0 0;0.0002 0;0.0004 0;0.0006 0;0.0008 0;0.001 0]  x3=[0 0;0.0002 0;0.0004 0;0.0006 0;0.0008 0;0.001 0]  x4=[0 0;0.0002 0;0.0004 0;0.0006 0;0.0008 0;0.001 0]  x5=0.001  Measurements=None
  Line_8 : powerlib/Elements/Distributed Parameters Line  DialogController=POWERSYS.PowerSysDialog  SystemSampleTime=-1  Phases=1  Frequency=60  Resistance=R(8)*1000  Inductance=L(8)*1000  Capacitance=C(8)*1000  Length=Len/(10*1000); % 10 sections in this subsystem  x1=[0 0;0.0002 0;0.0004 0;0.0006 0;0.0008 0;0.001 0]  x2=[0 0;0.0002 0;0.0004 0;0.0006 0;0.0008 0;0.001 0]  x3=[0 0;0.0002 0;0.0004 0;0.0006 0;0.0008 0;0.001 0]  x4=[0 0;0.0002 0;0.0004 0;0.0006 0;0.0008 0;0.001 0]  x5=0.001  Measurements=None
  Line_9 : powerlib/Elements/Distributed Parameters Line  DialogController=POWERSYS.PowerSysDialog  SystemSampleTime=-1  Phases=1  Frequency=60  Resistance=R(9)*1000  Inductance=L(9)*1000  Capacitance=C(9)*1000  Length=Len/(10*1000); % 10 sections in this subsystem  x1=[0 0;0.0002 0;0.0004 0;0.0006 0;0.0008 0;0.001 0]  x2=[0 0;0.0002 0;0.0004 0;0.0006 0;0.0008 0;0.001 0]  x3=[0 0;0.0002 0;0.0004 0;0.0006 0;0.0008 0;0.001 0]  x4=[0 0;0.0002 0;0.0004 0;0.0006 0;0.0008 0;0.001 0]  x5=0.001  Measurements=None
  Mux : Mux  Inputs=10
  VC{1..10} (10 alike) : powerlib/Measurements/Voltage Measurement  DialogController=POWERSYS.PowerSysDialog  SystemSampleTime=-1  PhasorSimulation=off  OutputType=Complex  PSBequivalent=0
  Connection Port : PMIOPort  Tag=PMCPort  Port=1  Side=Left
  Connection Port1 : PMIOPort  Tag=PMCPort  Port=2  Side=Left
  Connection Port2 : PMIOPort  Tag=PMCPort  Port=3  Side=Right
  Connection Port3 : PMIOPort  Tag=PMCPort  Port=4  Side=Right
  Vc : Outport  OutDataType=fixdt(1, 16)  OutScaling=2^0
  wires:
  VC1/1 -> Mux/1
  VC10/1 -> Mux/10
  VC9/1 -> Mux/9
  VC8/1 -> Mux/8
  VC7/1 -> Mux/7
  VC6/1 -> Mux/6
  VC5/1 -> Mux/5
  VC4/1 -> Mux/4
  VC3/1 -> Mux/3
  VC2/1 -> Mux/2
  Mux/1 -> Vc/1
  connections:
  Connection Port1/RConn1 -- Connection Port3/RConn1 -- VC10/LConn2 -- VC9/LConn2 -- VC8/LConn2 -- VC7/LConn2 -- VC6/LConn2 -- VC5/LConn2 -- VC4/LConn2 -- VC3/LConn2 -- VC2/LConn2 -- VC1/LConn2
  Line_10/RConn1 -- Connection Port2/RConn1
  Connection Port/RConn1 -- Line_1/LConn1 -- VC1/LConn1
  Line_1/RConn1 -- Line_2/LConn1 -- VC2/LConn1
  Line_2/RConn1 -- Line_3/LConn1 -- VC3/LConn1
  Line_3/RConn1 -- Line_4/LConn1 -- VC4/LConn1
  Line_4/RConn1 -- Line_5/LConn1 -- VC5/LConn1
  Line_5/RConn1 -- Line_6/LConn1 -- VC6/LConn1
  Line_6/RConn1 -- Line_7/LConn1 -- VC7/LConn1
  Line_7/RConn1 -- Line_8/LConn1 -- VC8/LConn1
  Line_8/RConn1 -- Line_9/LConn1 -- VC9/LConn1
  Line_9/RConn1 -- Line_10/LConn1 -- VC10/LConn1

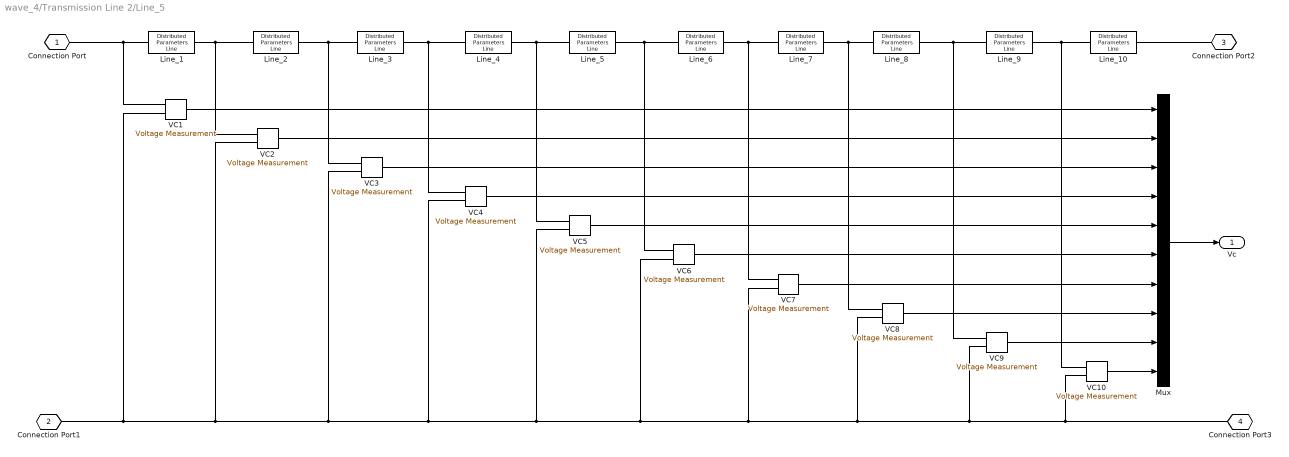
== system wave_4/Transmission Line 2/Line_5 ==
  Line_1 : powerlib/Elements/Distributed Parameters Line  DialogController=POWERSYS.PowerSysDialog  SystemSampleTime=-1  Phases=1  Frequency=60  Resistance=R(1)*1000  Inductance=L(1)*1000  Capacitance=C(1)*1000  Length=Len/(10*1000); % 10 sections in this subsystem  x1=[0 0;0.0002 0;0.0004 0;0.0006 0;0.0008 0;0.001 0]  x2=[0 0;0.0002 0;0.0004 0;0.0006 0;0.0008 0;0.001 0]  x3=[0 0;0.0002 0;0.0004 0;0.0006 0;0.0008 0;0.001 0]  x4=[0 0;0.0002 0;0.0004 0;0.0006 0;0.0008 0;0.001 0]  x5=0.001  Measurements=None
  Line_10 : powerlib/Elements/Distributed Parameters Line  DialogController=POWERSYS.PowerSysDialog  SystemSampleTime=-1  Phases=1  Frequency=60  Resistance=R(10)*1000  Inductance=L(10)*1000  Capacitance=C(10)*1000  Length=Len/(10*1000); % 10 sections in this subsystem  x1=[0 0;0.0002 0;0.0004 0;0.0006 0;0.0008 0;0.001 0]  x2=[0 0;0.0002 0;0.0004 0;0.0006 0;0.0008 0;0.001 0]  x3=[0 0;0.0002 0;0.0004 0;0.0006 0;0.0008 0;0.001 0]  x4=[0 0;0.0002 0;0.0004 0;0.0006 0;0.0008 0;0.001 0]  x5=0.001  Measurements=None
  Line_2 : powerlib/Elements/Distributed Parameters Line  DialogController=POWERSYS.PowerSysDialog  SystemSampleTime=-1  Phases=1  Frequency=60  Resistance=R(2)*1000  Inductance=L(2)*1000  Capacitance=C(2)*1000  Length=Len/(10*1000); % 10 sections in this subsystem  x1=[0 0;0.0002 0;0.0004 0;0.0006 0;0.0008 0;0.001 0]  x2=[0 0;0.0002 0;0.0004 0;0.0006 0;0.0008 0;0.001 0]  x3=[0 0;0.0002 0;0.0004 0;0.0006 0;0.0008 0;0.001 0]  x4=[0 0;0.0002 0;0.0004 0;0.0006 0;0.0008 0;0.001 0]  x5=0.001  Measurements=None
  Line_3 : powerlib/Elements/Distributed Parameters Line  DialogController=POWERSYS.PowerSysDialog  SystemSampleTime=-1  Phases=1  Frequency=60  Resistance=R(3)*1000  Inductance=L(3)*1000  Capacitance=C(3)*1000  Length=Len/(10*1000); % 10 sections in this subsystem  x1=[0 0;0.0002 0;0.0004 0;0.0006 0;0.0008 0;0.001 0]  x2=[0 0;0.0002 0;0.0004 0;0.0006 0;0.0008 0;0.001 0]  x3=[0 0;0.0002 0;0.0004 0;0.0006 0;0.0008 0;0.001 0]  x4=[0 0;0.0002 0;0.0004 0;0.0006 0;0.0008 0;0.001 0]  x5=0.001  Measurements=None
  Line_4 : powerlib/Elements/Distributed Parameters Line  DialogController=POWERSYS.PowerSysDialog  SystemSampleTime=-1  Phases=1  Frequency=60  Resistance=R(4)*1000  Inductance=L(4)*1000  Capacitance=C(4)*1000  Length=Len/(10*1000); % 10 sections in this subsystem  x1=[0 0;0.0002 0;0.0004 0;0.0006 0;0.0008 0;0.001 0]  x2=[0 0;0.0002 0;0.0004 0;0.0006 0;0.0008 0;0.001 0]  x3=[0 0;0.0002 0;0.0004 0;0.0006 0;0.0008 0;0.001 0]  x4=[0 0;0.0002 0;0.0004 0;0.0006 0;0.0008 0;0.001 0]  x5=0.001  Measurements=None
  Line_5 : powerlib/Elements/Distributed Parameters Line  DialogController=POWERSYS.PowerSysDialog  SystemSampleTime=-1  Phases=1  Frequency=60  Resistance=R(5)*1000  Inductance=L(5)*1000  Capacitance=C(5)*1000  Length=Len/(10*1000); % 10 sections in this subsystem  x1=[0 0;0.0002 0;0.0004 0;0.0006 0;0.0008 0;0.001 0]  x2=[0 0;0.0002 0;0.0004 0;0.0006 0;0.0008 0;0.001 0]  x3=[0 0;0.0002 0;0.0004 0;0.0006 0;0.0008 0;0.001 0]  x4=[0 0;0.0002 0;0.0004 0;0.0006 0;0.0008 0;0.001 0]  x5=0.001  Measurements=None
  Line_6 : powerlib/Elements/Distributed Parameters Line  DialogController=POWERSYS.PowerSysDialog  SystemSampleTime=-1  Phases=1  Frequency=60  Resistance=R(6)*1000  Inductance=L(6)*1000  Capacitance=C(6)*1000  Length=Len/(10*1000); % 10 sections in this subsystem  x1=[0 0;0.0002 0;0.0004 0;0.0006 0;0.0008 0;0.001 0]  x2=[0 0;0.0002 0;0.0004 0;0.0006 0;0.0008 0;0.001 0]  x3=[0 0;0.0002 0;0.0004 0;0.0006 0;0.0008 0;0.001 0]  x4=[0 0;0.0002 0;0.0004 0;0.0006 0;0.0008 0;0.001 0]  x5=0.001  Measurements=None
  Line_7 : powerlib/Elements/Distributed Parameters Line  DialogController=POWERSYS.PowerSysDialog  SystemSampleTime=-1  Phases=1  Frequency=60  Resistance=R(7)*1000  Inductance=L(7)*1000  Capacitance=C(7)*1000  Length=Len/(10*1000); % 10 sections in this subsystem  x1=[0 0;0.0002 0;0.0004 0;0.0006 0;0.0008 0;0.001 0]  x2=[0 0;0.0002 0;0.0004 0;0.0006 0;0.0008 0;0.001 0]  x3=[0 0;0.0002 0;0.0004 0;0.0006 0;0.0008 0;0.001 0]  x4=[0 0;0.0002 0;0.0004 0;0.0006 0;0.0008 0;0.001 0]  x5=0.001  Measurements=None
  Line_8 : powerlib/Elements/Distributed Parameters Line  DialogController=POWERSYS.PowerSysDialog  SystemSampleTime=-1  Phases=1  Frequency=60  Resistance=R(8)*1000  Inductance=L(8)*1000  Capacitance=C(8)*1000  Length=Len/(10*1000); % 10 sections in this subsystem  x1=[0 0;0.0002 0;0.0004 0;0.0006 0;0.0008 0;0.001 0]  x2=[0 0;0.0002 0;0.0004 0;0.0006 0;0.0008 0;0.001 0]  x3=[0 0;0.0002 0;0.0004 0;0.0006 0;0.0008 0;0.001 0]  x4=[0 0;0.0002 0;0.0004 0;0.0006 0;0.0008 0;0.001 0]  x5=0.001  Measurements=None
  Line_9 : powerlib/Elements/Distributed Parameters Line  DialogController=POWERSYS.PowerSysDialog  SystemSampleTime=-1  Phases=1  Frequency=60  Resistance=R(9)*1000  Inductance=L(9)*1000  Capacitance=C(9)*1000  Length=Len/(10*1000); % 10 sections in this subsystem  x1=[0 0;0.0002 0;0.0004 0;0.0006 0;0.0008 0;0.001 0]  x2=[0 0;0.0002 0;0.0004 0;0.0006 0;0.0008 0;0.001 0]  x3=[0 0;0.0002 0;0.0004 0;0.0006 0;0.0008 0;0.001 0]  x4=[0 0;0.0002 0;0.0004 0;0.0006 0;0.0008 0;0.001 0]  x5=0.001  Measurements=None
  Mux : Mux  Inputs=10
  VC{1..10} (10 alike) : powerlib/Measurements/Voltage Measurement  DialogController=POWERSYS.PowerSysDialog  SystemSampleTime=-1  PhasorSimulation=off  OutputType=Complex  PSBequivalent=0
  Connection Port : PMIOPort  Tag=PMCPort  Port=1  Side=Left
  Connection Port1 : PMIOPort  Tag=PMCPort  Port=2  Side=Left
  Connection Port2 : PMIOPort  Tag=PMCPort  Port=3  Side=Right
  Connection Port3 : PMIOPort  Tag=PMCPort  Port=4  Side=Right
  Vc : Outport  OutDataType=fixdt(1, 16)  OutScaling=2^0
  wires:
  Mux/1 -> Vc/1
  VC2/1 -> Mux/2
  VC3/1 -> Mux/3
  VC4/1 -> Mux/4
  VC5/1 -> Mux/5
  VC6/1 -> Mux/6
  VC7/1 -> Mux/7
  VC8/1 -> Mux/8
  VC9/1 -> Mux/9
  VC10/1 -> Mux/10
  VC1/1 -> Mux/1
  connections:
  VC10/LConn1 -- Line_10/LConn1 -- Line_9/RConn1
  VC9/LConn1 -- Line_9/LConn1 -- Line_8/RConn1
  VC8/LConn1 -- Line_8/LConn1 -- Line_7/RConn1
  VC7/LConn1 -- Line_7/LConn1 -- Line_6/RConn1
  VC6/LConn1 -- Line_6/LConn1 -- Line_5/RConn1
  VC5/LConn1 -- Line_5/LConn1 -- Line_4/RConn1
  VC4/LConn1 -- Line_4/LConn1 -- Line_3/RConn1
  VC3/LConn1 -- Line_3/LConn1 -- Line_2/RConn1
  VC2/LConn1 -- Line_2/LConn1 -- Line_1/RConn1
  VC1/LConn1 -- Line_1/LConn1 -- Connection Port/RConn1
  Line_10/RConn1 -- Connection Port2/RConn1
  VC1/LConn2 -- VC2/LConn2 -- VC3/LConn2 -- VC4/LConn2 -- VC5/LConn2 -- VC6/LConn2 -- VC7/LConn2 -- VC8/LConn2 -- VC9/LConn2 -- VC10/LConn2 -- Connection Port3/RConn1 -- Connection Port1/RConn1

== matlab function Wave Visualizer /Line Section Tap Voltage ==
  data: y input double; t input double; Line_Length input double; t_VSWR input double
function wave_plot(y, t, Line_Length,t_VSWR)
%#eml
eml.extrinsic('plot');
eml.extrinsic('axis');
eml.extrinsic('drawnow');
eml.extrinsic('xlabel');
eml.extrinsic('ylabel');
eml.extrinsic('text');
eml.extrinsic('sprintf');
eml.extrinsic('gcf');
eml.extrinsic('Peakfind')

persistent h;
persistent ht;
persistent x;
persistent maxPeak
persistent minPeak
persistent PeakData
persistent VSWR
persistent Dfac
persistent Dcount

if isempty(h) 
 x=((0:(length(y)-1))*Line_Length/50);   % 50 sub lines per Transmission Line Block  
 h=plot(x,y); axis([0,max(x), -1,1]); drawnow;
 set(gcf,'position',[50,50,500,250]);
 xlabel('X Position in Meters'); ylabel('Voltage');
 ht=text(0,-.5,sprintf('  t= %7.4f',t));
 maxPeak=-10;
 minPeak= 10;
 VSWR=0;
 PeakData=zeros(1,3);
 Dfac=10;  % update text readout every Dfac times
 Dcount=0;  % 
else
 set(h,'ydata',y); drawnow;
 if t>t_VSWR
    % Estimate VSWR on first transmission line after 
    % the first reflections should have arrived
    % the final value of the simulation run should be the best accuracy
    PeakData= Peakfind(x(1:50),y(1:50)',1);   
    maxPeak = max(maxPeak,max(PeakData(:,3)));
    minPeak = min(minPeak,min(PeakData(:,3)));
    VSWR=maxPeak/minPeak; % the maximum voltage on the line divided by the minimum should be the VSWR
    if VSWR>70
        VSWR=inf; % anything over 70:1 is essentially infinity VSWR
    end
     if Dcount==0
       set(ht,'string',sprintf('  t= %7.4f,   Line 1 VSWR=%5.1f:1',t,VSWR));
     end;
     
 else
     if Dcount==0
       set(ht,'string',sprintf('  t= %7.4f',t)); 
     end;
 end
    Dcount=Dcount+1;
    if Dcount>=Dfac
        Dcount=0;
    end;
end;
